simulink model "DRISHTI_Engine_Twin"  (R2026a)
settings: Solver=ode45  StopTime=120  MaxStep=0.01
libraries: simulink x2
settings Model: Creator=bhanu  LastModifiedBy=bhanu

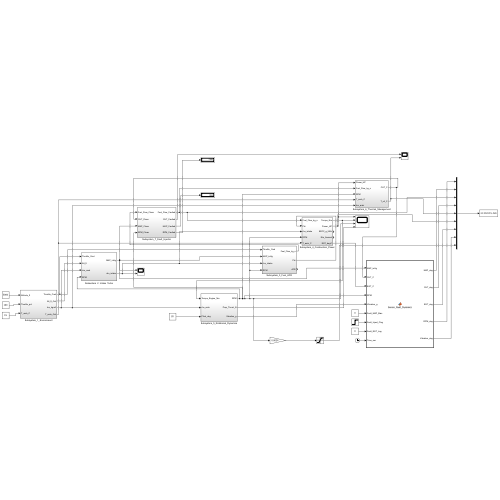
[thumbnail: Simulink's stored preview of the top-level diagram]
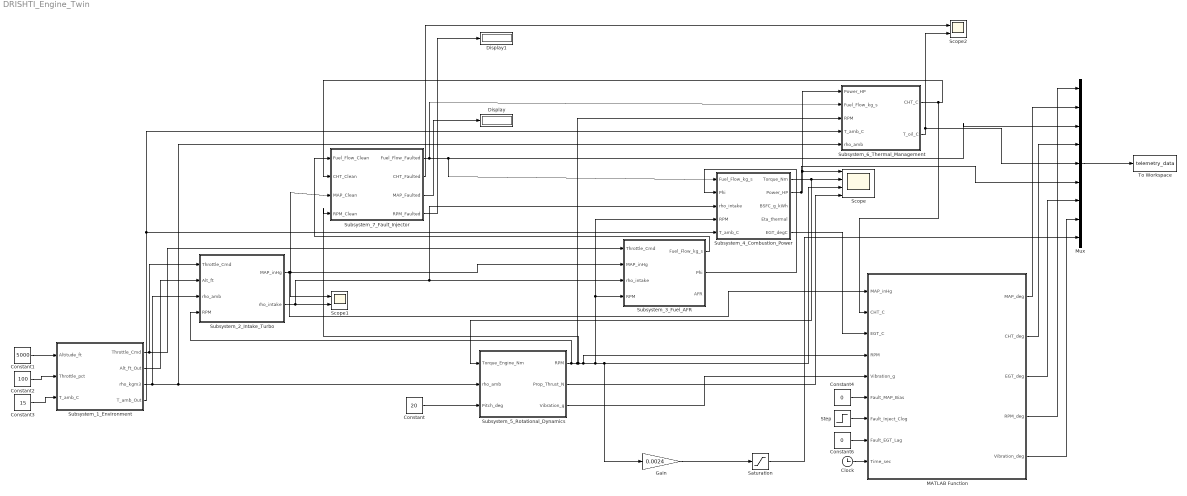
== system DRISHTI_Engine_Twin ==
  Clock : Clock
  Constant : Constant  Value=20
  Constant1 : Constant  Value=5000
  Constant2 : Constant  Value=100
  Constant3 : Constant  Value=15
  Constant4 : Constant  Value=0
  Constant6 : Constant  Value=0
  Display : Display
  Display1 : Display
  Gain : Gain  Gain=0.0024
  MATLAB Function : MATLAB Function  TreatAsAtomicUnit=on
  Mux : Mux  Inputs=9
  Saturation : Saturate  UpperLimit=14.2  LowerLimit=11.5
  Scope : Scope  NumInputPorts=4
      settings: ActiveDisplayYMinimum=-385.61866189035277  ActiveDisplayYMaximum=3705.9661135117153
  Scope1 : Scope  NumInputPorts=2
      settings: ActiveDisplayYMinimum=-1  ActiveDisplayYMaximum=1
  Scope2 : Scope  NumInputPorts=2
      settings: ActiveDisplayYMinimum=-20.819965273226813  ActiveDisplayYMaximum=175.12092867346072  DataLoggingVariableName=ScopeData2
  Step : Step  Time=10  SampleTime=0
  Subsystem_1_Environment : Subsystem
  Subsystem_2_Intake_Turbo : Subsystem
  Subsystem_3_Fuel_AFR : Subsystem
  Subsystem_4_Combustion_Power : Subsystem
  Subsystem_5_Rotational_Dynamics : Subsystem
  Subsystem_6_Thermal_Management : Subsystem
  Subsystem_7_Fault_Injector : Subsystem
  To Workspace : ToWorkspace  VariableName=telemetry_data  SampleTime=-1
  wires:
  Subsystem_1_Environment/1(Throttle_Cmd) -> Subsystem_3_Fuel_AFR/1(Throttle_Cmd), Subsystem_2_Intake_Turbo/1(Throttle_Cmd)
  Subsystem_1_Environment/2(Alt_ft_Out) -> Subsystem_2_Intake_Turbo/2(Alt_ft)
  Constant1/1 -> Subsystem_1_Environment/1(Altitude_ft)
  Constant2/1 -> Subsystem_1_Environment/2(Throttle_pct)
  Constant3/1 -> Subsystem_1_Environment/3(T_amb_C)
  Subsystem_2_Intake_Turbo/1(MAP_inHg) -> MATLAB Function/1(MAP_inHg), Subsystem_3_Fuel_AFR/2(MAP_inHg), Subsystem_7_Fault_Injector/3(MAP_Clean), Scope1/1
  Subsystem_1_Environment/3(rho_kgm3) -> Subsystem_6_Thermal_Management/5(rho_amb), Subsystem_5_Rotational_Dynamics/2(rho_amb), Subsystem_2_Intake_Turbo/3(rho_amb)
  Subsystem_7_Fault_Injector/2(CHT_Faulted) -> Scope2/1
  Subsystem_7_Fault_Injector/1(Fuel_Flow_Faulted) -> Mux/3, Subsystem_4_Combustion_Power/1(Fuel_Flow_kg_s), Subsystem_6_Thermal_Management/2(Fuel_Flow_kg_s)
  Subsystem_1_Environment/4(T_amb_Out) -> Subsystem_6_Thermal_Management/4(T_amb_C), Subsystem_4_Combustion_Power/5(T_amb_C)
  Subsystem_4_Combustion_Power/5(EGT_degC) -> MATLAB Function/3(EGT_C)
  Subsystem_2_Intake_Turbo/2(rho_intake) -> Subsystem_3_Fuel_AFR/3(rho_intake), Subsystem_4_Combustion_Power/3(rho_intake), Scope1/2
  Constant/1 -> Subsystem_5_Rotational_Dynamics/3(Pitch_deg)
  Subsystem_7_Fault_Injector/3(MAP_Faulted) -> Display/1
  Mux/1 -> To Workspace/1
  Subsystem_7_Fault_Injector/4(RPM_Faulted) -> Display1/1
  Subsystem_5_Rotational_Dynamics/2(Prop_Thrust_N) -> Scope/4
  Subsystem_5_Rotational_Dynamics/1(RPM) -> Subsystem_2_Intake_Turbo/4(RPM), MATLAB Function/4(RPM), Scope/3, Gain/1, Subsystem_4_Combustion_Power/4(RPM), Subsystem_3_Fuel_AFR/4(RPM), Subsystem_7_Fault_Injector/4(RPM_Clean), Subsystem_6_Thermal_Management/3(RPM)
  Subsystem_5_Rotational_Dynamics/3(Vibration_g) -> MATLAB Function/5(Vibration_g)
  Subsystem_3_Fuel_AFR/1(Fuel_Flow_kg_s) -> Subsystem_7_Fault_Injector/1(Fuel_Flow_Clean)
  Subsystem_4_Combustion_Power/1(Torque_Nm) -> Subsystem_5_Rotational_Dynamics/1(Torque_Engine_Nm), Scope/2
  Subsystem_3_Fuel_AFR/2(Phi) -> Subsystem_4_Combustion_Power/2(Phi)
  Gain/1 -> Saturation/1
  Subsystem_4_Combustion_Power/2(Power_HP) -> Scope/1, Subsystem_6_Thermal_Management/1(Power_HP), Mux/6
  Saturation/1 -> Mux/9
  Subsystem_6_Thermal_Management/2(T_oil_C) -> Mux/5, Scope2/2
  Subsystem_6_Thermal_Management/1(CHT_C) -> MATLAB Function/2(CHT_C), Subsystem_7_Fault_Injector/2(CHT_Clean)
  Constant4/1 -> MATLAB Function/6(Fault_MAP_Bias)
  Step/1 -> MATLAB Function/7(Fault_Inject_Clog)
  Constant6/1 -> MATLAB Function/8(Fault_EGT_Lag)
  Clock/1 -> MATLAB Function/9(Time_sec)
  MATLAB Function/5(Vibration_deg) -> Mux/8
  MATLAB Function/3(EGT_deg) -> Mux/7
  MATLAB Function/2(CHT_deg) -> Mux/4
  MATLAB Function/4(RPM_deg) -> Mux/1
  MATLAB Function/1(MAP_deg) -> Mux/2

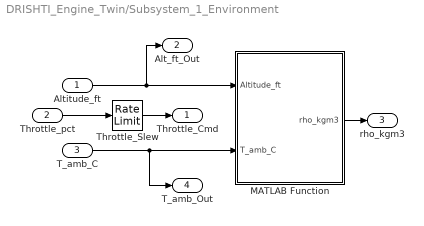
== system DRISHTI_Engine_Twin/Subsystem_1_Environment ==
  Altitude_ft : Inport
  Throttle_pct : Inport  Port=2
  T_amb_C : Inport  Port=3
  MATLAB Function : MATLAB Function  TreatAsAtomicUnit=on
  Throttle_Slew : RateLimiter  RisingSlewLimit=50  FallingSlewLimit=-50  SampleTimeMode=inherited
  Throttle_Cmd : Outport
  Alt_ft_Out : Outport  Port=2
  rho_kgm3 : Outport  Port=3
  T_amb_Out : Outport  Port=4
  wires:
  Throttle_pct/1 -> Throttle_Slew/1
  Throttle_Slew/1 -> Throttle_Cmd/1
  Altitude_ft/1 -> Alt_ft_Out/1, MATLAB Function/1(Altitude_ft)
  MATLAB Function/1(rho_kgm3) -> rho_kgm3/1
  T_amb_C/1 -> T_amb_Out/1, MATLAB Function/2(T_amb_C)

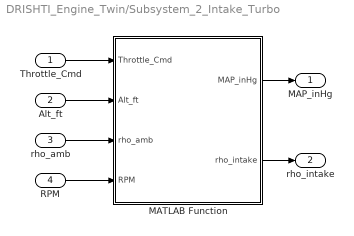
== system DRISHTI_Engine_Twin/Subsystem_2_Intake_Turbo ==
  Throttle_Cmd : Inport
  Alt_ft : Inport  Port=2
  rho_amb : Inport  Port=3
  RPM : Inport  Port=4
  MATLAB Function : MATLAB Function  TreatAsAtomicUnit=on
  MAP_inHg : Outport
  rho_intake : Outport  Port=2
  wires:
  Throttle_Cmd/1 -> MATLAB Function/1(Throttle_Cmd)
  Alt_ft/1 -> MATLAB Function/2(Alt_ft)
  rho_amb/1 -> MATLAB Function/3(rho_amb)
  MATLAB Function/1(MAP_inHg) -> MAP_inHg/1
  MATLAB Function/2(rho_intake) -> rho_intake/1
  RPM/1 -> MATLAB Function/4(RPM)

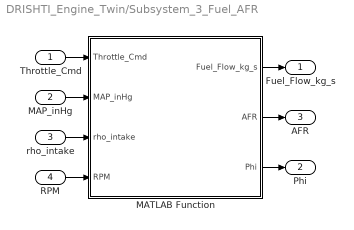
== system DRISHTI_Engine_Twin/Subsystem_3_Fuel_AFR ==
  Throttle_Cmd : Inport
  MAP_inHg : Inport  Port=2
  rho_intake : Inport  Port=3
  RPM : Inport  Port=4
  MATLAB Function : MATLAB Function  TreatAsAtomicUnit=on
  Fuel_Flow_kg_s : Outport
  Phi : Outport  Port=2
  AFR : Outport  Port=3
  wires:
  Throttle_Cmd/1 -> MATLAB Function/1(Throttle_Cmd)
  MAP_inHg/1 -> MATLAB Function/2(MAP_inHg)
  rho_intake/1 -> MATLAB Function/3(rho_intake)
  RPM/1 -> MATLAB Function/4(RPM)
  MATLAB Function/1(Fuel_Flow_kg_s) -> Fuel_Flow_kg_s/1
  MATLAB Function/2(AFR) -> AFR/1
  MATLAB Function/3(Phi) -> Phi/1

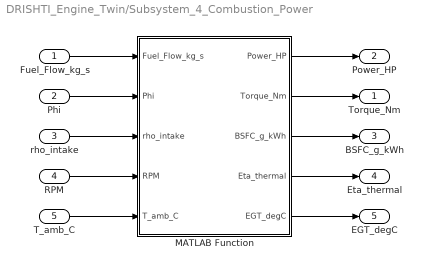
== system DRISHTI_Engine_Twin/Subsystem_4_Combustion_Power ==
  Fuel_Flow_kg_s : Inport
  Phi : Inport  Port=2
  rho_intake : Inport  Port=3
  RPM : Inport  Port=4
  T_amb_C : Inport  Port=5
  MATLAB Function : MATLAB Function  TreatAsAtomicUnit=on
  Torque_Nm : Outport
  Power_HP : Outport  Port=2
  BSFC_g_kWh : Outport  Port=3
  Eta_thermal : Outport  Port=4
  EGT_degC : Outport  Port=5
  wires:
  Fuel_Flow_kg_s/1 -> MATLAB Function/1(Fuel_Flow_kg_s)
  Phi/1 -> MATLAB Function/2(Phi)
  rho_intake/1 -> MATLAB Function/3(rho_intake)
  RPM/1 -> MATLAB Function/4(RPM)
  T_amb_C/1 -> MATLAB Function/5(T_amb_C)
  MATLAB Function/1(Power_HP) -> Power_HP/1
  MATLAB Function/2(Torque_Nm) -> Torque_Nm/1
  MATLAB Function/3(BSFC_g_kWh) -> BSFC_g_kWh/1
  MATLAB Function/4(Eta_thermal) -> Eta_thermal/1
  MATLAB Function/5(EGT_degC) -> EGT_degC/1

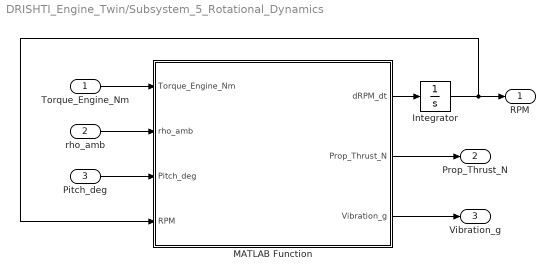
== system DRISHTI_Engine_Twin/Subsystem_5_Rotational_Dynamics ==
  Torque_Engine_Nm : Inport
  rho_amb : Inport  Port=2
  Pitch_deg : Inport  Port=3
  Integrator : Integrator  InitialCondition=1400
  MATLAB Function : MATLAB Function  TreatAsAtomicUnit=on
  RPM : Outport
  Prop_Thrust_N : Outport  Port=2
  Vibration_g : Outport  Port=3
  wires:
  Torque_Engine_Nm/1 -> MATLAB Function/1(Torque_Engine_Nm)
  rho_amb/1 -> MATLAB Function/2(rho_amb)
  Pitch_deg/1 -> MATLAB Function/3(Pitch_deg)
  MATLAB Function/2(Prop_Thrust_N) -> Prop_Thrust_N/1
  MATLAB Function/1(dRPM_dt) -> Integrator/1
  Integrator/1 -> RPM/1, MATLAB Function/4(RPM)
  MATLAB Function/3(Vibration_g) -> Vibration_g/1

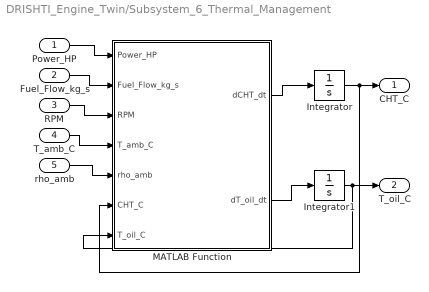
== system DRISHTI_Engine_Twin/Subsystem_6_Thermal_Management ==
  Power_HP : Inport
  Fuel_Flow_kg_s : Inport  Port=2
  RPM : Inport  Port=3
  T_amb_C : Inport  Port=4
  rho_amb : Inport  Port=5
  Integrator : Integrator  InitialCondition=15
  Integrator1 : Integrator  InitialCondition=15
  MATLAB Function : MATLAB Function  TreatAsAtomicUnit=on
  CHT_C : Outport
  T_oil_C : Outport  Port=2
  wires:
  MATLAB Function/1(dCHT_dt) -> Integrator/1
  MATLAB Function/2(dT_oil_dt) -> Integrator1/1
  Integrator/1 -> MATLAB Function/6(CHT_C), CHT_C/1
  Integrator1/1 -> MATLAB Function/7(T_oil_C), T_oil_C/1
  Power_HP/1 -> MATLAB Function/1(Power_HP)
  Fuel_Flow_kg_s/1 -> MATLAB Function/2(Fuel_Flow_kg_s)
  RPM/1 -> MATLAB Function/3(RPM)
  T_amb_C/1 -> MATLAB Function/4(T_amb_C)
  rho_amb/1 -> MATLAB Function/5(rho_amb)

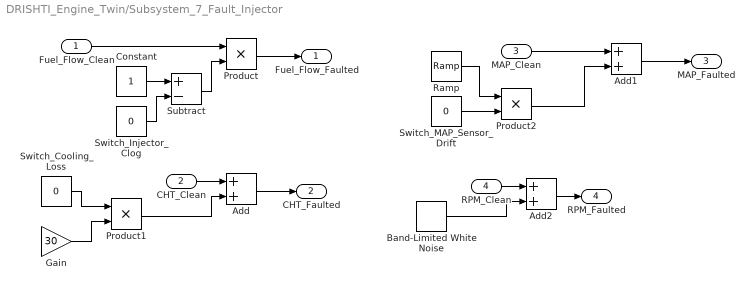
== system DRISHTI_Engine_Twin/Subsystem_7_Fault_Injector ==
  Fuel_Flow_Clean : Inport
  CHT_Clean : Inport  Port=2
  MAP_Clean : Inport  Port=3
  RPM_Clean : Inport  Port=4
  Add : Sum
  Add1 : Sum
  Add2 : Sum
  Band-Limited White Noise : simulink/Sources/Band-Limited White Noise  Cov=10  Ts=0.01  seed=[23341]
  Constant : Constant
  Gain : Gain  Gain=30
  Product : Product
  Product1 : Product
  Product2 : Product
  Ramp : simulink/Sources/Ramp  slope=0.05  start=0  InitialOutput=0
  Subtract : Sum  Inputs=+-
  Switch_Cooling_Loss : Constant  Value=0
  Switch_Injector_Clog : Constant  Value=0
  Switch_MAP_Sensor_Drift : Constant  Value=0
  Fuel_Flow_Faulted : Outport
  CHT_Faulted : Outport  Port=2
  MAP_Faulted : Outport  Port=3
  RPM_Faulted : Outport  Port=4
  wires:
  Constant/1 -> Subtract/1
  Switch_Injector_Clog/1 -> Subtract/2
  Fuel_Flow_Clean/1 -> Product/1
  Subtract/1 -> Product/2
  Product/1 -> Fuel_Flow_Faulted/1
  Switch_Cooling_Loss/1 -> Product1/1
  Gain/1 -> Product1/2
  CHT_Clean/1 -> Add/1
  Product1/1 -> Add/2
  Add/1 -> CHT_Faulted/1
  Ramp/1 -> Product2/1
  Switch_MAP_Sensor_Drift/1 -> Product2/2
  MAP_Clean/1 -> Add1/1
  Product2/1 -> Add1/2
  Add1/1 -> MAP_Faulted/1
  RPM_Clean/1 -> Add2/1
  Band-Limited White Noise/1 -> Add2/2
  Add2/1 -> RPM_Faulted/1

== matlab function DRISHTI_Engine_Twin/Subsystem_2_Intake_Turbo/MATLAB Function ==
  settings: updateMethod=DISCRETE
  data: Throttle_Cmd input; MAP_inHg output; Alt_ft input; rho_amb input; rho_intake output; RPM input
function [MAP_inHg, rho_intake] = Turbo_Intake_Dynamics(Throttle_Cmd, Alt_ft, rho_amb, RPM)
% =========================================================================
% ROTAX 914 UL/F - HIGH-FIDELITY TURBO & INTAKE DYNAMICS
% Includes:
% 1. International Standard Atmosphere (ISA) Pressure Derivation
% 2. Non-linear Wastegate Actuator Limits & Rate-Limited Lag Dynamics
% 3. Compressor Map Pressure Ratio Saturation Limits
% 4. Isentropic Compressor Temperature Rise & Intercooler Effectiveness
% 5. Real-Time Intake Manifold Air Density Calculation
% =========================================================================

    % 1. Ambient Pressure Calculation from ISA Model (inHg)
    P0_inHg = 29.92;
    if Alt_ft <= 36089
        P_amb = P0_inHg * (1.0 - 6.8755e-6 * Alt_ft)^5.2559;
    else
        P_amb = 6.68 * exp(-(Alt_ft - 36089) / 20800);
    end

    % 2. Wastegate Actuator Target MAP (Rotax 914 OEM Envelope)
    % Sea-level continuous boost limit: 35.4 inHg | Takeoff boost limit (5 min): 39.9 inHg
    throttle_norm = min(max(Throttle_Cmd / 100.0, 0.0), 1.0);
    MAP_target = P_amb + (39.9 - P_amb) * (throttle_norm^1.2);

    % 3. First-Order Wastegate Actuator Dynamic Lag
    persistent MAP_prev
    if isempty(MAP_prev)
        MAP_prev = P_amb;
    end
    
    tau_wastegate = 0.15; % Wastegate dynamic time constant (seconds)
    dt = 0.01;            % Fixed simulation time step
    
    % Low-pass discrete filtering for pneumatic valve lag
    MAP_filtered = MAP_prev + (dt / (tau_wastegate + dt)) * (MAP_target - MAP_prev);
    MAP_prev = MAP_filtered;

    % 4. Turbocharger Compressor Saturation Limits
    % Rotax 914 Garrett Turbocharger Max Pressure Ratio = 1.68
    PR_max = 1.68;
    MAP_achievable = P_amb * PR_max;
    MAP_inHg = min(MAP_filtered, MAP_achievable);

    % 5. Thermodynamics: Compressor Temperature & Intercooler Effectiveness
    gamma = 1.4;              % Ratio of specific heats for air
    eta_compressor = 0.72;    % Compressor Isentropic Efficiency (72%)
    PR_actual = max(1.0, MAP_inHg / max(P_amb, 0.1));

    % Temperature rise across turbo compressor stage
    T_amb_K = 288.15 - 0.0019812 * Alt_ft;
    T_comp_out = T_amb_K * (1.0 + (1.0 / eta_compressor) * (PR_actual^((gamma - 1.0) / gamma) - 1.0));

    % Intercooler thermal exchanger (65% cooling effectiveness)
    eta_intercooler = 0.65;
    T_airbox_K = T_comp_out - eta_intercooler * (T_comp_out - T_amb_K);

    % 6. Ideal Gas Law for Manifold Air Density (rho_intake in kg/m^3)
    R_air = 287.058;                     % Specific gas constant for air [J/(kg*K)]
    P_pascal = MAP_inHg * 3386.39;        % Convert inHg to Pascals
    rho_intake = P_pascal / (R_air * T_airbox_K);

end

== matlab function DRISHTI_Engine_Twin/Subsystem_1_Environment/MATLAB Function ==
  data: Altitude_ft input; rho_kgm3 output; T_amb_C input
function rho_kgm3 = ISA_Air_Density(Altitude_ft, T_amb_C)
% Calculates ambient air density based on altitude and temperature
% Inputs: Altitude_ft (ft), T_amb_C (°C)
% Output: rho_kgm3 (kg/m^3)

% Conversions
alt_m = Altitude_ft * 0.3048; % Convert feet to meters
T_K = T_amb_C + 273.15;       % Convert °C to Kelvin

% ISA Constants
g = 9.80665;     % Acceleration due to gravity (m/s^2)
R = 287.058;     % Specific gas constant for dry air (J/(kg*K))
L = 0.0065;      % Temperature lapse rate (K/m)
T0 = 288.15;     % Sea level standard temperature (K)
P0 = 101325;     % Sea level standard pressure (Pa)

% Pressure calculation considering lapse rate
P = P0 * (1 - (L * alt_m) / T0)^(g / (R * L));

% Density using Ideal Gas Law
rho_kgm3 = P / (R * T_K);
end

== matlab function DRISHTI_Engine_Twin/Subsystem_3_Fuel_AFR/MATLAB Function ==
  data: Throttle_Cmd input; Fuel_Flow_kg_s output; MAP_inHg input; rho_intake input; RPM input; AFR output; Phi output
function [Fuel_Flow_kg_s, AFR, Phi] = Fuel_System_Dynamics(Throttle_Cmd, MAP_inHg, rho_intake, RPM)
% Rotax 914 Carburetor & Fuel Injection Model
% Calculates Fuel Mass Flow (kg/s), Air-Fuel Ratio (AFR), and Equivalence Ratio (Phi)

% --- Engine Displacement & Constants ---
V_d = 0.001211; % Rotax 914 displacement in m^3 (1211 cc)
AFR_stoich = 14.7; % Stoichiometric AFR for standard gasoline

% 1. Air Mass Flow Rate Calculation (Speed-Density Method)
% Volumetric efficiency estimate (Eta_v) based on RPM and MAP
eta_v = 0.82 + 0.08 * (MAP_inHg / 38.4) - 0.05 * (RPM / 5800)^2;
eta_v = max(0.65, min(0.95, eta_v));

% Intake mass flow rate of air (kg/s)
m_dot_air = (rho_intake * V_d * (RPM / 60) * 0.5) * eta_v;

% 2. Target AFR Mapping (Enrichment at high power / takeoff boost)
if Throttle_Cmd > 100
    target_AFR = 11.8; % Rich mixture for cooling & detonation suppression during overboost
elseif Throttle_Cmd > 75
    target_AFR = 12.5; % Power enrichment
else
    target_AFR = 14.0; % Lean cruise economy
end

% 3. Fuel Mass Flow Rate (kg/s)
Fuel_Flow_kg_s = m_dot_air / target_AFR;

% 4. Actual AFR and Equivalence Ratio (Phi = AFR_stoich / AFR)
AFR = target_AFR;
Phi = AFR_stoich / AFR;

end

== matlab function DRISHTI_Engine_Twin/Subsystem_4_Combustion_Power/MATLAB Function ==
  data: Fuel_Flow_kg_s input; Power_HP output; Phi input; rho_intake input; RPM input; T_amb_C input; Torque_Nm output; BSFC_g_kWh output; Eta_thermal output; EGT_degC output
function [Power_HP, Torque_Nm, BSFC_g_kWh, Eta_thermal, EGT_degC] = Combustion_Power_Dynamics(Fuel_Flow_kg_s, Phi, rho_intake, RPM, T_amb_C)
% =========================================================================
% ROTAX 914 UL/F - HIGH-FIDELITY COMBUSTION & POWER DYNAMICS
% Includes:
% 1. Wiebe Combustion Efficiency Curve vs. Equivalence Ratio (Phi)
% 2. Chen-Flynn Engine Friction Model (FMEP to Mechanical Power Loss)
% 3. Indicated vs Brake Power Balance
% 4. Dynamic Exhaust Gas Temperature (EGT) Energy Balance
% 5. Real-Time BSFC and Brake Torque Calculation
% =========================================================================

    % --- Rotax 914 Engine Constants ---
    LHV_gasoline = 43.5e6;    % Lower Heating Value of gasoline (J/kg)
    V_d = 0.001211;           % Engine displacement volume (1211 cc = 0.001211 m^3)
    P_max_rated_HP = 115.0;   % Rated Max Power (HP)
    
    % 1. Wiebe Function Equivalence Ratio (Phi) Efficiency
    % Optimal combustion efficiency occurs near stoichiometric (Phi ~ 0.98 - 1.05)
    if Phi > 1.0
        % Rich mixture: Incomplete combustion penalty
        eta_comb = 0.98 - 0.22 * (Phi - 1.0)^1.35;
    else
        % Lean mixture: Flame propagation slowdown penalty
        eta_comb = 0.98 - 0.28 * (1.0 - Phi)^1.2;
    end
    eta_comb = max(0.50, min(0.98, eta_comb));

    % 2. Indicated Thermal Efficiency (Otto Cycle Basis)
    r_c = 9.0;               % Compression Ratio of Rotax 914
    gamma = 1.35;            % Ratio of specific heats for combustion gases
    eta_otto = 1.0 - (1.0 / (r_c^(gamma - 1.0)));
    
    % Air intake density correction factor
    rho_std = 1.225;         % Standard sea-level air density (kg/m^3)
    density_factor = min(1.2, max(0.6, rho_intake / rho_std));
    
    Eta_thermal = eta_otto * eta_comb * (0.88 + 0.12 * density_factor);

    % 3. Total Thermal Heat Input & Indicated Power
    Q_dot_in = Fuel_Flow_kg_s * LHV_gasoline;   % Fuel Energy Rate (Watts)
    P_indicated_W = Q_dot_in * Eta_thermal;      % Indicated Power (Watts)

    % 4. Chen-Flynn Mechanical Friction Model (FMEP)
    % FMEP (Pascals) = C1 + C2*P_max + C3*Mean_Piston_Speed
    N_rps = RPM / 60.0;
    stroke = 0.061;                              % Stroke length (61 mm)
    Sp = 2.0 * stroke * N_rps;                   % Mean Piston Speed (m/s)
    
    FMEP_Pa = (0.4e5) + (0.005 * P_indicated_W / max(1.0, V_d * N_rps)) + (0.12e5 * Sp);
    P_friction_W = FMEP_Pa * V_d * (N_rps / 2.0); % 4-stroke cycle friction loss

    % 5. Net Brake Power & Shaft Torque
    Brake_Power_W = max(0.0, P_indicated_W - P_friction_W);
    Power_HP = Brake_Power_W / 745.7;

    omega = (RPM * 2.0 * pi) / 60.0;
    if omega > 10.0
        Torque_Nm = Brake_Power_W / omega;
    else
        Torque_Nm = 0.0;
    end

    % 6. Brake Specific Fuel Consumption (BSFC) [g/kWh]
    if Power_HP > 2.0
        Fuel_Flow_g_h = Fuel_Flow_kg_s * 3600.0 * 1000.0;
        Power_kW = Power_HP * 0.7457;
        BSFC_g_kWh = Fuel_Flow_g_h / Power_kW;
    else
        BSFC_g_kWh = 0.0;
    end

    % 7. Thermodynamic Exhaust Gas Temperature (EGT in deg C)
    % Unburned fuel in rich mixtures lowers EGT; lean burning raises EGT up to peak
    T_ambient = T_amb_C + 273.15;
    Q_unburned_W = Q_dot_in * (1.0 - eta_comb);
    Cp_exhaust = 1150.0;                          % Exhaust gas heat capacity [J/(kg*K)]
    
    % Total exhaust mass flow rate (air + fuel)
    m_dot_exhaust = max(0.005, Fuel_Flow_kg_s * (1.0 + 14.7 / max(0.5, Phi)));
    
    % Baseline combustion temperature + unburned enthalpy effects
    Delta_T_exhaust = (P_indicated_W * 0.55 + Q_unburned_W * 0.20) / (m_dot_exhaust * Cp_exhaust);
    EGT_K = T_ambient + Delta_T_exhaust;
    
    EGT_degC = min(950.0, max(T_amb_C, EGT_K - 273.15));

end

== matlab function DRISHTI_Engine_Twin/Subsystem_5_Rotational_Dynamics/MATLAB Function ==
  data: Torque_Engine_Nm input; dRPM_dt output; rho_amb input; Pitch_deg input; RPM input; Prop_Thrust_N output; Vibration_g output
function [dRPM_dt, Prop_Thrust_N, Vibration_g] = Rotational_Prop_Dynamics(Torque_Engine_Nm, rho_amb, Pitch_deg, RPM)
% =========================================================================
% ROTAX 914 UL/F - HIGH-FIDELITY ROTATIONAL DYNAMICS & PROP LOAD MODEL
% Outputs:
% 1. dRPM_dt (RPM/s) - Crankshaft Acceleration
% 2. Prop_Thrust_N (N) - Aerodynamic Propeller Thrust Output
% 3. Vibration_g (g) - Engine & Prop Unbalance Vibration Level
% =========================================================================

    % --- Rotax 914 Mechanical Parameters ---
    gear_ratio = 2.43;      % Gearbox reduction ratio (2.43:1)
    eta_gearbox = 0.96;     % Gearbox mechanical efficiency
    D_prop = 1.72;          % Propeller diameter (meters)
    J_total = 0.285;        % Total reflected rotational inertia (kg*m^2)

    % 1. Propeller Shaft Speed & Aerodynamic Load
    n_prop = max(0.0, (RPM / 60.0) / gear_ratio); % Propeller rev/s
    
    % Non-linear Torque Coefficient (C_q) scaled by variable pitch angle
    pitch_norm = max(0.2, Pitch_deg / 20.0);
    K_p = 0.0125;
    C_q = K_p * (pitch_norm^1.15);
    
    % Aerodynamic Propeller Load Torque reflected to crankshaft
    Torque_Prop_Absorbed = C_q * rho_amb * (n_prop^2) * (D_prop^5);
    Torque_Prop_Crankshaft = Torque_Prop_Absorbed / (gear_ratio * eta_gearbox);

    % 2. Net Torque Balance & Rotational Acceleration
    Net_Torque_Nm = Torque_Engine_Nm - Torque_Prop_Crankshaft;
    domega_dt = Net_Torque_Nm / J_total;
    dRPM_dt = domega_dt * (60.0 / (2.0 * pi));

    % 3. Aerodynamic Thrust Output
    % Non-linear Thrust Coefficient (C_t)
    C_t = C_q * (3.45 - 0.25 * pitch_norm);
    Prop_Thrust_N = max(0.0, C_t * rho_amb * (n_prop^2) * (D_prop^4));

    % 4. Engine & Shaft Vibration Model (1st & 2nd Order Harmonics)
    % Base mechanical imbalance scaling + rotational speed squared
    rpm_norm = max(0.0, RPM) / 5800.0;
    vibe_baseline = 0.15 + 1.2 * (rpm_norm^2);
    
    % High-frequency imbalance component (g-units)
    vibe_noise = 0.08 * sin(2.0 * pi * (RPM / 60.0) * 0.01);
    Vibration_g = min(10.0, max(0.0, vibe_baseline + vibe_noise));

end

== matlab function DRISHTI_Engine_Twin/Subsystem_6_Thermal_Management/MATLAB Function ==
  data: Power_HP input; dCHT_dt output; Fuel_Flow_kg_s input; RPM input; T_amb_C input; rho_amb input; dT_oil_dt output; CHT_C input; T_oil_C input
function [dCHT_dt, dT_oil_dt] = Thermal_Dynamics(Power_HP, Fuel_Flow_kg_s, RPM, T_amb_C, rho_amb, CHT_C, T_oil_C)
% =========================================================================
% ROTAX 914 UL/F - HIGH-FIDELITY THERMAL DYNAMICS MODEL
% Outputs temperature derivatives (dCHT/dt, dT_oil/dt) in °C/s
% Includes:
% 1. Continuous CHT-to-Oil Convective Heat Transfer Exchange
% 2. Dynamic Ram-Air Speed & Air Density Scaled Convective Cooling
% 3. Engine RPM-Driven Oil Circulation Rate & Radiator Dissipation
% =========================================================================

    % --- Thermal Mass Constants ---
    m_cht = 18.5;            % Effective thermal mass of cylinder head assembly (kg)
    cp_alu = 890.0;          % Specific heat capacity of aluminum alloy (J/kg*K)
    m_oil = 3.5;             % Total oil capacity (kg)
    cp_oil = 1900.0;         % Specific heat capacity of synthetic engine oil (J/kg*K)
    LHV_gasoline = 43.5e6;   % Lower Heating Value (J/kg)

    % 1. Total Heat Rejected to Metal Structure & Coolant
    Q_dot_total = Fuel_Flow_kg_s * LHV_gasoline;
    Power_Watts = max(0.0, Power_HP * 745.7);
    Q_dot_waste = max(0.0, Q_dot_total - Power_Watts); % Non-mechanical thermal energy

    % Energy distribution breakdown: ~28% directly into cylinder heads, ~12% friction to oil
    Q_dot_to_CHT = 0.28 * Q_dot_waste;
    Q_dot_friction_oil = (0.05 * Power_Watts) + (1200.0 * (max(RPM, 0.0) / 5800.0)^2);

    % 2. Convective Air Cooling & Internal Heat Exchange
    % Airspeed scales dynamically with atmospheric density ratio
    rho_std = 1.225;
    V_airspeed = 38.0 * sqrt(rho_std / max(0.3, rho_amb)); % Dynamic flight velocity (m/s)
    h_air = 18.0 + 3.2 * sqrt(V_airspeed);                 % Convective heat transfer coeff

    % Head-to-Oil Heat Transfer (Oil jacket cooling path)
    h_head_oil = 45.0; % Inter-component heat exchange coefficient (W/K)
    Q_dot_head_to_oil = h_head_oil * (CHT_C - T_oil_C);

    % Heat dissipation to surrounding ambient air
    Q_dot_cht_cool = h_air * 0.85 * (CHT_C - T_amb_C);
    
    % Oil cooler heat dissipation (RPM-driven mechanical oil pump flow)
    h_radiator = h_air * 0.45 + 0.12 * RPM;
    Q_dot_oil_cool = h_radiator * (T_oil_C - T_amb_C);

    % 3. Differential Heat Rate Equations (°C/s)
    dCHT_dt = (Q_dot_to_CHT - Q_dot_head_to_oil - Q_dot_cht_cool) / (m_cht * cp_alu);
    dT_oil_dt = (Q_dot_friction_oil + Q_dot_head_to_oil - Q_dot_oil_cool) / (m_oil * cp_oil);

end

== matlab function DRISHTI_Engine_Twin/MATLAB Function ==
  settings: updateMethod=DISCRETE
  data: MAP_inHg input; MAP_deg output; CHT_C input; EGT_C input; RPM input; Vibration_g input; Fault_MAP_Bias input; Fault_Inject_Clog input; Fault_EGT_Lag input; Time_sec input; CHT_deg output; EGT_deg output; RPM_deg output; Vibration_deg output
function [MAP_deg, CHT_deg, EGT_deg, RPM_deg, Vibration_deg] = Sensor_Fault_Dynamics(...
    MAP_inHg, CHT_C, EGT_C, RPM, Vibration_g, ...
    Fault_MAP_Bias, Fault_Inject_Clog, Fault_EGT_Lag, Time_sec)
% =========================================================================
% ROTAX 914 DIGITAL TWIN - SENSOR NOISE & FAULT INJECTION LAYER
% Models sensor degradation, white noise, thermocouple thermal lag,
% and physical system faults (injector clogging, pressure sensor drift).
% =========================================================================

    % --- 1. Manifold Absolute Pressure Sensor (MAP Drift Fault) ---
    % Normal sensor noise (~0.05 inHg std dev)
    map_noise = 0.05 * sin(2*pi*15*Time_sec) + 0.02 * cos(2*pi*43*Time_sec);
    MAP_deg = max(0.0, MAP_inHg + map_noise + Fault_MAP_Bias);

    % --- 2. Cylinder Head Temperature Sensor (CHT Dynamics) ---
    % CHT thermistor white noise
    cht_noise = 0.15 * sin(2*pi*5*Time_sec);
    CHT_deg = max(0.0, CHT_C + cht_noise);

    % --- 3. Exhaust Gas Temperature (EGT Thermocouple Response Lag) ---
    % EGT thermocouples have a noticeable thermal lag (~0.8 sec time constant)
    persistent EGT_sensor_state
    if isempty(EGT_sensor_state)
        EGT_sensor_state = EGT_C;
    end
    
    tau_egt = 0.8; % Thermocouple thermal time constant
    if Fault_EGT_Lag > 0
        tau_egt = tau_egt * 3.0; % Triple the lag if sensor degraded
    end
    
    dt = 0.01;
    EGT_sensor_state = EGT_sensor_state + (dt / (tau_egt + dt)) * (EGT_C - EGT_sensor_state);
    egt_noise = 0.8 * sin(2*pi*8*Time_sec);
    EGT_deg = max(0.0, EGT_sensor_state + egt_noise);

    % --- 4. Engine Speed Sensor (Pick-up Optical Noise / Injector Clogging Fault) ---
    % Clogged injector creates power imbalance and RPM jitter
    clog_jitter = 0.0;
    if Fault_Inject_Clog > 0
        clog_jitter = 45.0 * sin(2*pi*12*Time_sec) * Fault_Inject_Clog;
    end
    rpm_noise = 3.0 * sin(2*pi*25*Time_sec);
    RPM_deg = max(0.0, RPM + rpm_noise + clog_jitter);

    % --- 5. Vibration Sensor (Accelerometer Noise) ---
    vibe_noise = 0.02 * sin(2*pi*60*Time_sec);
    % Fuel injector clogging increases engine unbalance vibration
    vibe_fault_effect = 0.8 * Fault_Inject_Clog;
    Vibration_deg = max(0.0, Vibration_g + vibe_noise + vibe_fault_effect);

end
